simulink model "Rider_Controls_InHardware_CAN_Enable"  (R2014b)
settings: configuration reference "Embedded_Configuration" (kept outside this file)
PreLoadFcn:
  | load('Embedded_Config.mat')
PostLoadFcn:
  | c2000demoscallback(1)
model workspace: external: MAT-File Embedded_Config.mat (data not in the file)
undefined symbols (not defined in the file or in its folder): canChannel
libraries: canmsglib x2, canlib x2, c280xlib x1
settings Model: Creator=The MathWorks Inc.  LastModifiedBy=Nathan

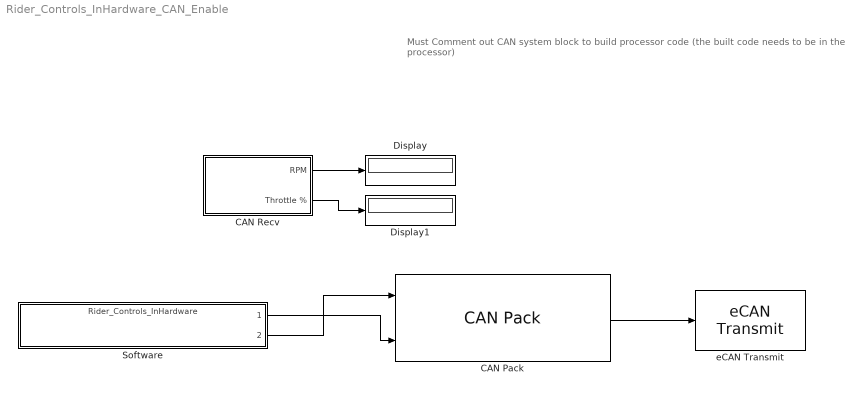
== system Rider_Controls_InHardware_CAN_Enable ==
  note: Must Comment out CAN system block
      | to build processor code
      | (the built code needs to be in the processor)
  CAN Pack : canmsglib/CAN Pack  CANdbFile=C:\Users\Nathan\Desktop\Git\EmbeddedCoderC2000\Rider_Controls\Rider_Controls_Debug.dbc  MsgList=Control_Input  MsgName=Control_Input  MsgIDType=Standard (11-bit identifier)  MsgIdentifier=0  MsgLength=8  SignalInfo=RPM$32$32$1$3$1$0$1$0$-100000$100000$#Throttle_percent$0$32$1$3$1$0$1$0$-1000$1000$#  NSignals=2  StartBits=str2num('[int32(32);int32(0)]')  SignalSizes=str2num('[int32(32);int32(32)]')  ByteOrders=str2num('[int32(1);int32(1)]')  DataTypes=str2num('[int32(3);int32(3)]')  MultiplexTypes=str2num('[int32(1);int32(1)]')  MultiplexValues=str2num('[double(0);double(0)]')  Factors=str2num('[double(1);double(1)]')  Offsets=str2num('[double(0);double(0)]')  Minimums=str2num('[double(-100000);double(-1000)]')  Maximums=str2num('[double(100000);double(1000)]')  Remote=off
      settings: DataFormat=CANdb specified signals
  CAN Recv : Subsystem
  Display : Display
  Display1 : Display
  Software : ModelReference  ModelNameDialog=Rider_Controls_InHardware.slx  SimulationMode=Normal  ModelReferenceVersion=1.100  CopyOfModelName=Rider_Controls_InHardware.slx  DefaultDataLogging=on
  eCAN Transmit : c280xlib/eCAN Transmit  chipFamily=C280x  useModule=eCAN_A  mailboxNo=1  messageID=0  messageType=Standard (11-bit identifier)  enableBlockingMode=off  postInterrupt=off  interruptLine=0
  wires:
  Software/1 -> CAN Pack/2
  CAN Pack/1 -> eCAN Transmit/1
  CAN Recv/1(RPM) -> Display/1
  Software/2 -> CAN Pack/1
  CAN Recv/2(Throttle %) -> Display1/1

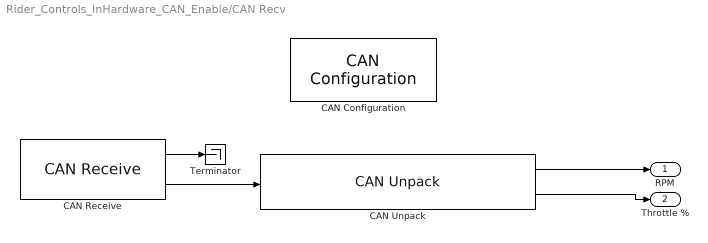
== system Rider_Controls_InHardware_CAN_Enable/CAN Recv ==
  CAN Configuration : canlib/CAN Configuration  BlockHandle=211.0007  DeviceMenu=Kvaser Eagle 1 (Channel 1)  Device=Kvaser Eagle 1 (Channel 1)  ObjConstructor=canChannel('Kvaser', 'Eagle 1', 1)  BusSpeed=500000  EnableBitParameters=off  SJW=1  TSEG1=4  TSEG2=3  NSamples=1  AckMode=Normal
  CAN Receive : canlib/CAN Receive  BlockHandle=213.0009  DeviceMenu=Kvaser Eagle 1 (Channel 1)  Device=Kvaser Eagle 1 (Channel 1)  ObjConstructor=canChannel('Kvaser', 'Eagle 1', 1)  EnableStandardIDsFilter=off  StandardIDs=0  EnableExtendedIDsFilter=off  ExtendedIDs=0  SampleTime=.01  MsgsPerTimestep=all  StdIDsCombo=Allow only  ExtIDsCombo=Block all  InternalFilterUpdateStatus=on
  CAN Unpack : canmsglib/CAN Unpack  CANdbFile=C:\Users\Nathan\Desktop\Git\EmbeddedCoderC2000\Rider_Controls\Rider_Controls_Debug.dbc  MsgList=Control_Input  MsgName=Control_Input  MsgIDType=Standard (11-bit identifier)  MsgIdentifier=0  MsgLength=8  SignalInfo=RPM$32$32$1$3$1$0$1$0$-100000$100000$#Throttle_percent$0$32$1$3$1$0$1$0$-1000$1000$#  NSignals=2  IDPort=off  TimestampPort=off  ErrorPort=off  RemotePort=off  LengthPort=off  StatusPort=off  StartBits=str2num('[int32(32);int32(0)]')  SignalSizes=str2num('[int32(32);int32(32)]')  ByteOrders=str2num('[int32(1);int32(1)]')  DataTypes=str2num('[int32(3);int32(3)]')  MultiplexTypes=str2num('[int32(1);int32(1)]')  MultiplexValues=str2num('[double(0);double(0)]')  Factors=str2num('[double(1);double(1)]')  Offsets=str2num('[double(0);double(0)]')  Minimums=str2num('[double(-100000);double(-1000)]')  Maximums=str2num('[double(100000);double(1000)]')
      settings: DataFormat=CANdb specified signals
  Terminator : Terminator
  RPM : Outport
  Throttle % : Outport  Port=2
  wires:
  CAN Unpack/1 -> RPM/1
  CAN Receive/2 -> CAN Unpack/1
  CAN Receive/1 -> Terminator/1
  CAN Unpack/2 -> Throttle %/1
